simulink model "projectile_2pm_ver1"  (Simulink 7.9)
settings: Solver=ode45  StartTime=0.0  StopTime=4  RelTol=1e-3
values from neighbouring files (symbols this model uses):
  CdC_m = 0.001731    [cmc_projectile_odegrads.m]    (also in cmc_projectile_odegrads2.m)
  g = 32.2    [cmc_projectile_odegrads.m]    (also in cmc_projectile_odegrads2.m)
  velx0 = cosd(theta)*vel0    [cmc_projectile_odegrads.m]    (also in cmc_projectile_odegrads2.m)
  vely0 = sind(theta)*vel0    [cmc_projectile_odegrads.m]    (also in cmc_projectile_odegrads2.m)
  x0 = 0    [Homework_3_ODEGRAD45.m]    (also in cmc_projectile_odegrads.m; cmc_projectile_odegrads2.m)
  y0 = 0.    (= 0)    [cmc_projectile_odegrads.m]    (also in cmc_projectile_odegrads2.m)
libraries: simulink x2
settings Model: Creator=cmc4177  LastModifiedBy=cmc4177

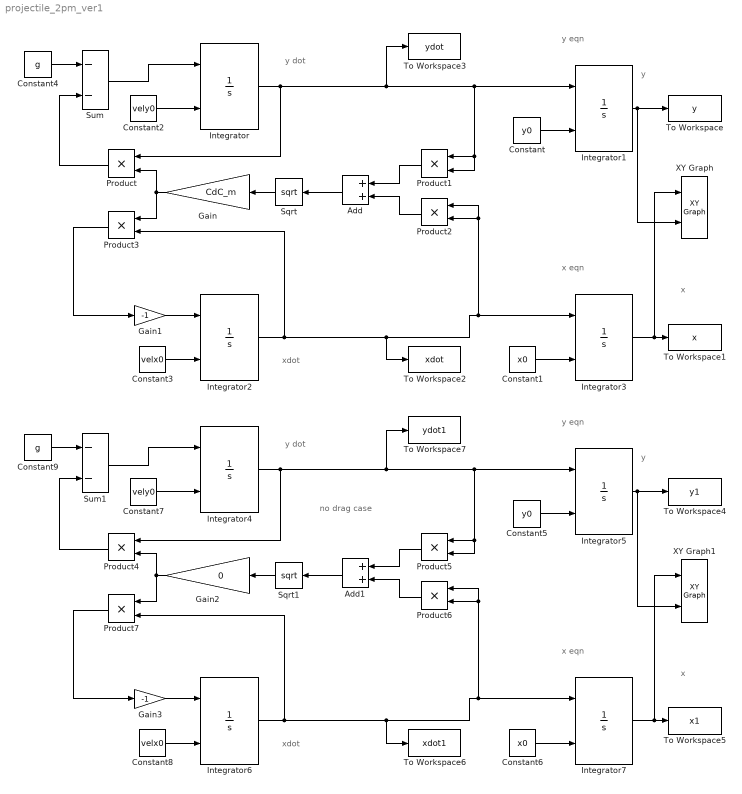
== system projectile_2pm_ver1 ==
  note: y eqn
  note: x eqn
  note: y dot
  note: y
  note: xdot
  note: x
  note: y eqn
  note: x eqn
  note: y dot
  note: y
  note: xdot
  note: x
  note: no drag case
  Add : Sum
  Add1 : Sum
  Constant : Constant  Value=y0
  Constant1 : Constant  Value=x0
  Constant2 : Constant  Value=vely0
  Constant3 : Constant  Value=velx0
  Constant4 : Constant  Value=g
  Constant5 : Constant  Value=y0
  Constant6 : Constant  Value=x0
  Constant7 : Constant  Value=vely0
  Constant8 : Constant  Value=velx0
  Constant9 : Constant  Value=g
  Gain : Gain  Gain=CdC_m
  Gain1 : Gain  Gain=-1
  Gain2 : Gain  Gain=0
  Gain3 : Gain  Gain=-1
  Integrator{,1..7} (8 alike) : Integrator  InitialConditionSource=external
  Product{,1..7} (8 alike) : Product  RndMeth=Zero
  Sqrt : Sqrt  SaturateOnIntegerOverflow=on
  Sqrt1 : Sqrt  SaturateOnIntegerOverflow=on
  Sum : Sum  Inputs=--
  Sum1 : Sum  Inputs=--
  To Workspace : ToWorkspace  VariableName=y  SampleTime=-1
  To Workspace1 : ToWorkspace  VariableName=x  SampleTime=-1
  To Workspace2 : ToWorkspace  VariableName=xdot  SampleTime=-1
  To Workspace3 : ToWorkspace  VariableName=ydot  SampleTime=-1
  To Workspace4 : ToWorkspace  VariableName=y1  SampleTime=-1
  To Workspace5 : ToWorkspace  VariableName=x1  SampleTime=-1
  To Workspace6 : ToWorkspace  VariableName=xdot1  SampleTime=-1
  To Workspace7 : ToWorkspace  VariableName=ydot1  SampleTime=-1
  XY Graph : simulink/Sinks/XY Graph  xmin=-1  xmax=1  ymin=-1  ymax=1  st=-1
  XY Graph1 : simulink/Sinks/XY Graph  xmin=-1  xmax=1  ymin=-1  ymax=1  st=-1
  wires:
  Integrator/1 -> Product/1, Integrator1/1, Product1/1, Product1/2, To Workspace3/1
  Constant/1 -> Integrator1/2
  Constant1/1 -> Integrator3/2
  Constant3/1 -> Integrator2/2
  Constant2/1 -> Integrator/2
  Integrator2/1 -> Product3/2, Integrator3/1, Product2/1, Product2/2, To Workspace2/1
  Product1/1 -> Add/1
  Product2/1 -> Add/2
  Add/1 -> Sqrt/1
  Sqrt/1 -> Gain/1
  Gain/1 -> Product/2, Product3/1
  Constant4/1 -> Sum/1
  Product/1 -> Sum/2
  Sum/1 -> Integrator/1
  Product3/1 -> Gain1/1
  Gain1/1 -> Integrator2/1
  Integrator1/1 -> XY Graph/2, To Workspace/1
  Integrator3/1 -> XY Graph/1, To Workspace1/1
  Integrator4/1 -> To Workspace7/1, Product5/2, Product5/1, Integrator5/1, Product4/1
  Constant5/1 -> Integrator5/2
  Constant6/1 -> Integrator7/2
  Constant8/1 -> Integrator6/2
  Constant7/1 -> Integrator4/2
  Integrator6/1 -> To Workspace6/1, Product6/2, Product6/1, Integrator7/1, Product7/2
  Product5/1 -> Add1/1
  Product6/1 -> Add1/2
  Add1/1 -> Sqrt1/1
  Sqrt1/1 -> Gain2/1
  Gain2/1 -> Product7/1, Product4/2
  Constant9/1 -> Sum1/1
  Product4/1 -> Sum1/2
  Sum1/1 -> Integrator4/1
  Product7/1 -> Gain3/1
  Gain3/1 -> Integrator6/1
  Integrator5/1 -> To Workspace4/1, XY Graph1/2
  Integrator7/1 -> To Workspace5/1, XY Graph1/1
